simulink model "Sensores_no_ideales"  (R2023a)
settings: Solver=VariableStepAuto  StartTime=0.0  StopTime=10.0  RelTol=1e-3
undefined symbols (not defined in the file or in its folder): omega_n, tau, zitta
settings Model: Creator=Juan  LastModifiedBy=Juan

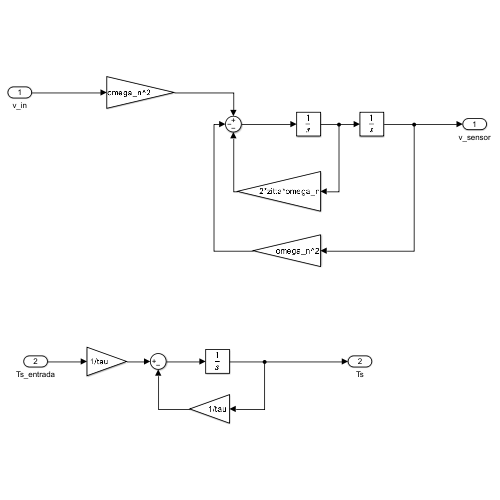
[thumbnail: Simulink's stored preview of the top-level diagram]
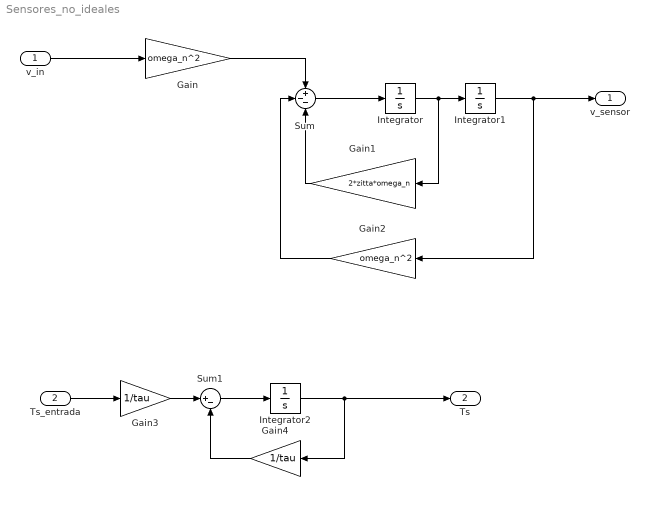
== system Sensores_no_ideales ==
  v_in : Inport
  Ts_entrada : Inport  Port=2
  Gain : Gain  Gain=omega_n^2
  Gain1 : Gain  Gain=2*zitta*omega_n
  Gain2 : Gain  Gain=omega_n^2
  Gain3 : Gain  Gain=1/tau
  Gain4 : Gain  Gain=1/tau
  Integrator : Integrator
  Integrator1 : Integrator
  Integrator2 : Integrator
  Sum : Sum  Inputs=+--
  Sum1 : Sum  Inputs=|+-
  v_sensor : Outport
  Ts : Outport  Port=2
  wires:
  v_in/1 -> Gain/1
  Gain/1 -> Sum/1
  Sum/1 -> Integrator/1
  Integrator/1 -> Gain1/1, Integrator1/1
  Integrator1/1 -> Gain2/1, v_sensor/1
  Gain2/1 -> Sum/2
  Gain1/1 -> Sum/3
  Gain3/1 -> Sum1/1
  Ts_entrada/1 -> Gain3/1
  Sum1/1 -> Integrator2/1
  Integrator2/1 -> Gain4/1, Ts/1
  Gain4/1 -> Sum1/2
